simulink model "SEIRS_3"  (R2024a)
settings: Solver=VariableStepAuto  StartTime=0.0  StopTime=2500  MaxStep=0.01  RelTol=1e-3
values from neighbouring files (symbols this model uses):
  x = S.x    [gsua_sample.m]
settings Model: Creator=carlo  LastModifiedBy=luism
settings DataIOCC: SaveOutput=off
settings RTWCC: GPUComputeCapability=3.5

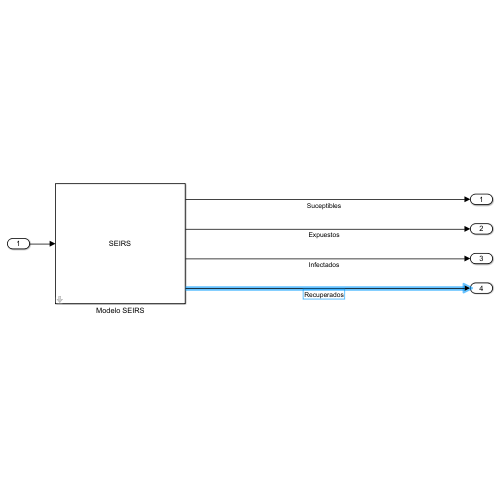
[thumbnail: Simulink's stored preview of the top-level diagram]
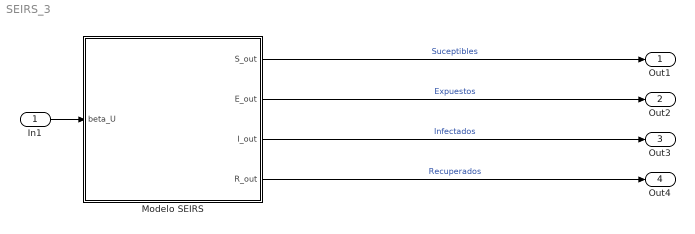
== system SEIRS_3 ==
  In1 : Inport
  Modelo SEIRS : Subsystem  mask{B=x(1), d=x(2), alpha=x(3), gamma=x(4), beta=x(5), nu=x(6), ci=[1-1e-6 1e-6 0 0]}
      mask prompts: ci "[S0 I0 R0 E0]"
      mask Display: disp('SEIRS');
  Out1 : Outport
  Out2 : Outport  Port=2
  Out3 : Outport  Port=3
  Out4 : Outport  Port=4
  wires:
  In1/1 -> Modelo SEIRS/1(beta_U)
  Modelo SEIRS/4(R_out) -> Out4/1  "Recuperados"
  Modelo SEIRS/3("I_out ") -> Out3/1  "Infectados"
  Modelo SEIRS/2(E_out) -> Out2/1  "Expuestos"
  Modelo SEIRS/1(S_out) -> Out1/1  "Suceptibles"

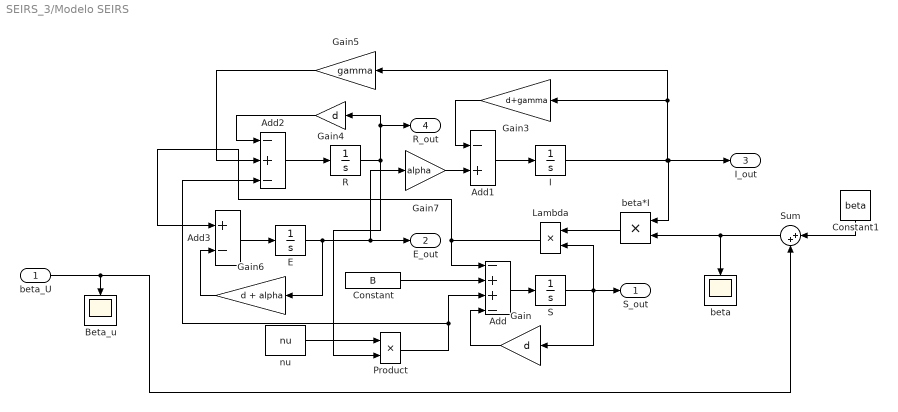
== system SEIRS_3/Modelo SEIRS ==
  beta_U : Inport
  Add : Sum  Inputs=-++-
  Add1 : Sum  Inputs=-+
  Add2 : Sum  Inputs=-+-
  Add3 : Sum  Inputs=+-
  Beta_u : Scope
  Constant : Constant  Value=B
  Constant1 : Constant  Value=beta
  E : Integrator  InitialCondition=ci(4)  LimitOutput=on  LowerSaturationLimit=0
  Gain : Gain  Gain=d
  Gain3 : Gain  Gain=d+gamma
  Gain4 : Gain  Gain=d
  Gain5 : Gain  Gain=gamma
  Gain6 : Gain  Gain=d + alpha
  Gain7 : Gain  Gain=alpha
  I : Integrator  InitialCondition=ci(2)  LimitOutput=on  LowerSaturationLimit=0
  Lambda : Product
  Product : Product
  R : Integrator  InitialCondition=ci(3)  LimitOutput=on  LowerSaturationLimit=0
  S : Integrator  InitialCondition=ci(1)  LimitOutput=on  LowerSaturationLimit=0
  Sum : Sum  Inputs=|++
  beta : Scope
  beta*I : Product
  nu : Constant  Value=nu
  S_out : Outport
  E_out : Outport  Port=2
  "I_out " : Outport  Port=3
  R_out : Outport  Port=4
  wires:
  Gain/1 -> Add/4
  Gain4/1 -> Add2/1
  Constant/1 -> Add/2
  I/1 -> beta*I/1, "I_out "/1, Gain5/1, Gain3/1
  Lambda/1 -> Add3/1, Add/1
  Add/1 -> S/1
  E/1 -> E_out/1, Gain7/1, Gain6/1
  S/1 -> S_out/1, Gain/1, Lambda/2
  Add3/1 -> E/1
  Gain3/1 -> Add1/1
  Gain5/1 -> Add2/2
  Gain6/1 -> Add3/2
  Add1/1 -> I/1
  R/1 -> Gain4/1, R_out/1, Product/2
  Add2/1 -> R/1
  Product/1 -> Add2/3, Add/3
  Gain7/1 -> Add1/2
  nu/1 -> Product/1
  beta*I/1 -> Lambda/1
  Sum/1 -> beta*I/2, beta/1
  Constant1/1 -> Sum/1
  beta_U/1 -> Sum/2, Beta_u/1
